simulink model "prob3"  (R2020b)
settings: Solver=VariableStepAuto  StartTime=0.0  StopTime=0.1  RelTol=1e-3
settings Model: Creator=DELL  LastModifiedBy=DELL

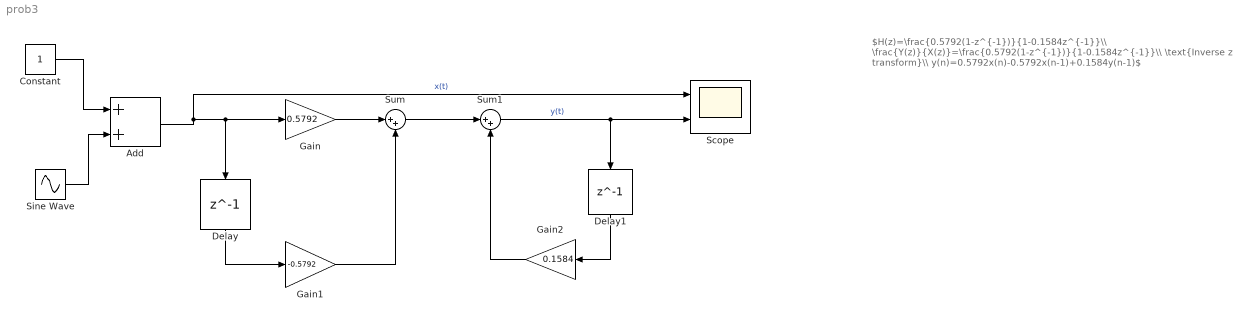
== system prob3 ==
  note: $H(z)=\frac{0.5792(1-z^{-1})}{1-0.1584z^{-1}}\\ \frac{Y(z)}{X(z)}=\frac{0.5792(1-z^{-1})}{1-0.1584z^{-1}}\\ \text{Inverse z transform}\\ y(n)=0.5792x(n)-0.5792x(n-1)+0.1584y(n-1)$
  Add : Sum
  Constant : Constant
  Delay : Delay  DelayLength=1
  Delay1 : Delay  DelayLength=1
  Gain : Gain  Gain=0.5792
  Gain1 : Gain  Gain=-0.5792
  Gain2 : Gain  Gain=0.1584
  Scope : Scope  NumInputPorts=2
  Sine Wave : Sin  Frequency=1000*2*pi  SampleTime=1/5000
  Sum : Sum  Inputs=|++
  Sum1 : Sum  Inputs=|++
  wires:
  Add/1 -> Scope/1, Gain/1, Delay/1  "x(t)"
  Delay/1 -> Gain1/1
  Gain/1 -> Sum/1
  Gain1/1 -> Sum/2
  Sum/1 -> Sum1/1
  Sum1/1 -> Scope/2, Delay1/1  "y(t)"
  Delay1/1 -> Gain2/1
  Gain2/1 -> Sum1/2
  Sine Wave/1 -> Add/2
  Constant/1 -> Add/1
